simulink model "main"  (R2024b)
settings: Solver=VariableStepAuto  StartTime=0.0  StopTime=0.1  RelTol=1e-3
settings Model: Creator=Admin  LastModifiedBy=Admin

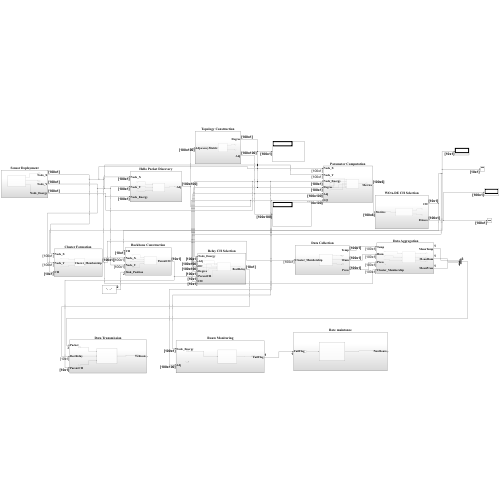
[thumbnail: Simulink's stored preview of the top-level diagram]
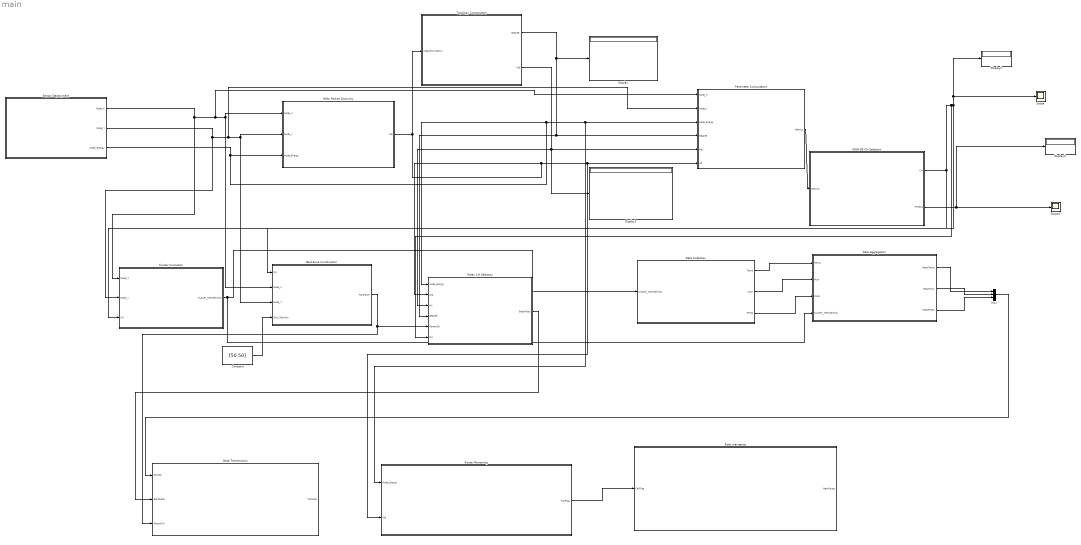
== system main ==
  " Data Aggregation" : Subsystem
  " Data Collection" : Subsystem
  " Route Monitoring" : Subsystem
  Backbone Construction : Subsystem
  Cluster Formation : Subsystem
  Constant : Constant  Value=[50 50]
  Data Transmission : Subsystem
  Display{,1..3} (4 alike) : Display
  Hello Packet Discovery : Subsystem
  Mux : Mux  Inputs=3
  Parameter Computation : Subsystem
  Relay CH Selection : Subsystem
  Rote maintance : Subsystem
  Scope : Scope
  Scope1 : Scope
  Sensor Deployment : Subsystem
  Topology Construction : Subsystem
  WOA-DE CH Selection : Subsystem
  wires:
  Sensor Deployment/2(Node_Y) -> Cluster Formation/2(Node_Y), Parameter Computation/2(Node_Y), Backbone Construction/3(Node_Y), Hello Packet Discovery/2(Node_Y)
  Sensor Deployment/3(Node_Energy) -> Parameter Computation/3(Node_Energy), " Route Monitoring"/1(Node_Energy), Relay CH Selection/1(Node_Energy), Hello Packet Discovery/3(Node_Energy)
  Hello Packet Discovery/1(Adj) -> Parameter Computation/6(LQ), " Route Monitoring"/2(Adj), Relay CH Selection/2(Adj), Topology Construction/1(AdjacencyMatrix)
  Topology Construction/2(Adj) -> Parameter Computation/5(Adj), Relay CH Selection/3(HC), Display1/1
  Sensor Deployment/1(Node_X) -> Cluster Formation/1(Node_X), Backbone Construction/2(Node_X), Hello Packet Discovery/1(Node_X), Parameter Computation/1(Node_X)
  Topology Construction/1(Degree) -> Parameter Computation/4(Degree), Relay CH Selection/4(Degree), Display/1
  Parameter Computation/1(Metrics) -> WOA-DE CH Selection/1(Metrics)
  WOA-DE CH Selection/2(Fitness) -> Display3/1, Scope1/1
  WOA-DE CH Selection/1(CH) -> Relay CH Selection/6(CH), Display2/1, Scope/1, Backbone Construction/1(CH), Cluster Formation/3(CH)
  Constant/1 -> Backbone Construction/4(Sink_Position)
  Backbone Construction/1(ParentCH) -> Data Transmission/3(ParentCH), Relay CH Selection/5(ParentCH)
  Cluster Formation/1(Cluster_Membership) -> " Data Aggregation"/4(Cluster_Membership), " Data Collection"/1(Cluster_Membership)
  " Data Collection"/1(Temp) -> " Data Aggregation"/1(Temp)
  " Data Collection"/2(Hum) -> " Data Aggregation"/2(Hum)
  " Data Collection"/3(Press) -> " Data Aggregation"/3(Press)
  " Data Aggregation"/3(MeanPress) -> Mux/3
  " Data Aggregation"/2(MeanHum) -> Mux/2
  " Data Aggregation"/1(MeanTemp) -> Mux/1
  Mux/1 -> Data Transmission/1(Packet)
  Relay CH Selection/1(BestRelay) -> Data Transmission/2(BestRelay)
  " Route Monitoring"/1(FailFlag) -> Rote maintance/1(FailFlag)

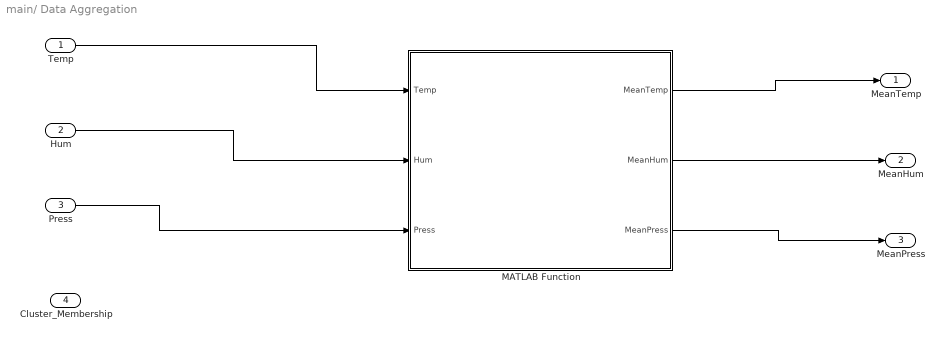
== system main/ Data Aggregation ==
  Temp : Inport
  Hum : Inport  Port=2
  Press : Inport  Port=3
  Cluster_Membership : Inport  Port=4
  MATLAB Function : MATLAB Function  TreatAsAtomicUnit=on
  MeanTemp : Outport
  MeanHum : Outport  Port=2
  MeanPress : Outport  Port=3
  wires:
  Temp/1 -> MATLAB Function/1(Temp)
  Hum/1 -> MATLAB Function/2(Hum)
  Press/1 -> MATLAB Function/3(Press)
  MATLAB Function/1(MeanTemp) -> MeanTemp/1
  MATLAB Function/2(MeanHum) -> MeanHum/1
  MATLAB Function/3(MeanPress) -> MeanPress/1

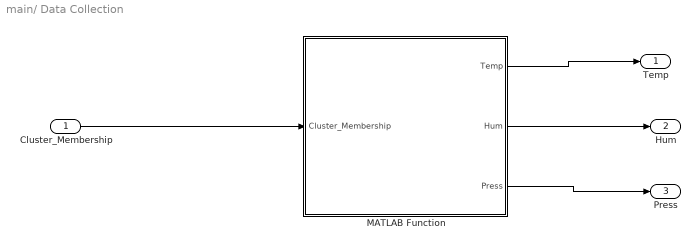
== system main/ Data Collection ==
  Cluster_Membership : Inport
  MATLAB Function : MATLAB Function  TreatAsAtomicUnit=on
  Temp : Outport
  Hum : Outport  Port=2
  Press : Outport  Port=3
  wires:
  Cluster_Membership/1 -> MATLAB Function/1(Cluster_Membership)
  MATLAB Function/1(Temp) -> Temp/1
  MATLAB Function/2(Hum) -> Hum/1
  MATLAB Function/3(Press) -> Press/1

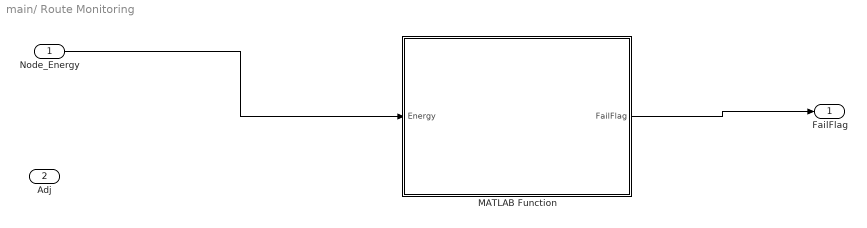
== system main/ Route Monitoring ==
  Node_Energy : Inport
  Adj : Inport  Port=2
  MATLAB Function : MATLAB Function  TreatAsAtomicUnit=on
  FailFlag : Outport
  wires:
  Node_Energy/1 -> MATLAB Function/1(Energy)
  MATLAB Function/1(FailFlag) -> FailFlag/1

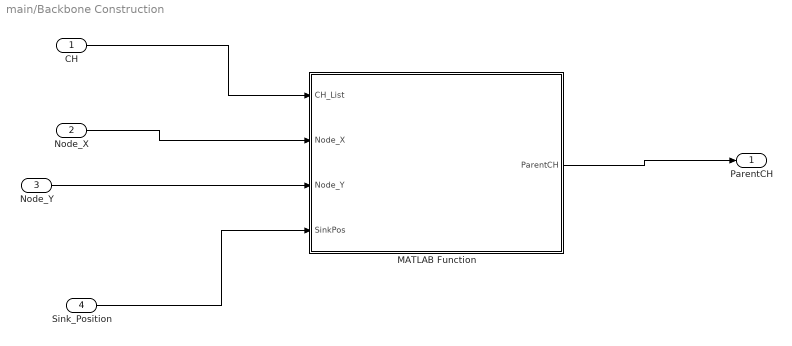
== system main/Backbone Construction ==
  CH : Inport
  Node_X : Inport  Port=2
  Node_Y : Inport  Port=3
  Sink_Position : Inport  Port=4
  MATLAB Function : MATLAB Function  TreatAsAtomicUnit=on
  ParentCH : Outport
  wires:
  CH/1 -> MATLAB Function/1(CH_List)
  Node_X/1 -> MATLAB Function/2(Node_X)
  Node_Y/1 -> MATLAB Function/3(Node_Y)
  Sink_Position/1 -> MATLAB Function/4(SinkPos)
  MATLAB Function/1(ParentCH) -> ParentCH/1

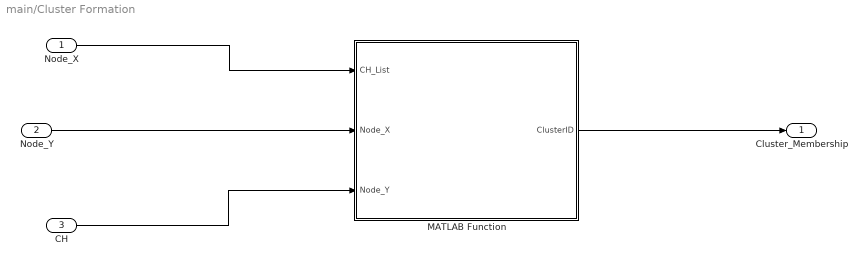
== system main/Cluster Formation ==
  Node_X : Inport
  Node_Y : Inport  Port=2
  CH : Inport  Port=3
  MATLAB Function : MATLAB Function  TreatAsAtomicUnit=on
  Cluster_Membership : Outport
  wires:
  Node_X/1 -> MATLAB Function/1(CH_List)
  Node_Y/1 -> MATLAB Function/2(Node_X)
  CH/1 -> MATLAB Function/3(Node_Y)
  MATLAB Function/1(ClusterID) -> Cluster_Membership/1

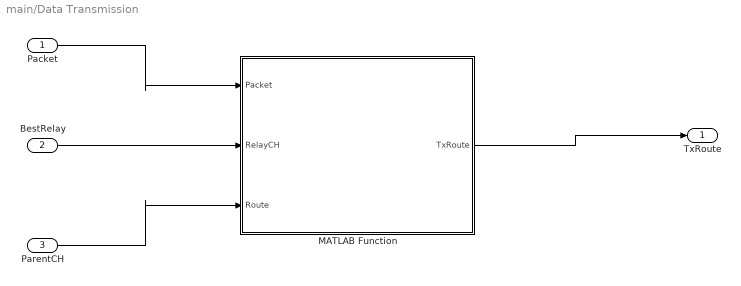
== system main/Data Transmission ==
  Packet : Inport
  BestRelay : Inport  Port=2
  ParentCH : Inport  Port=3
  MATLAB Function : MATLAB Function  TreatAsAtomicUnit=on
  TxRoute : Outport
  wires:
  Packet/1 -> MATLAB Function/1(Packet)
  BestRelay/1 -> MATLAB Function/2(RelayCH)
  ParentCH/1 -> MATLAB Function/3(Route)
  MATLAB Function/1(TxRoute) -> TxRoute/1

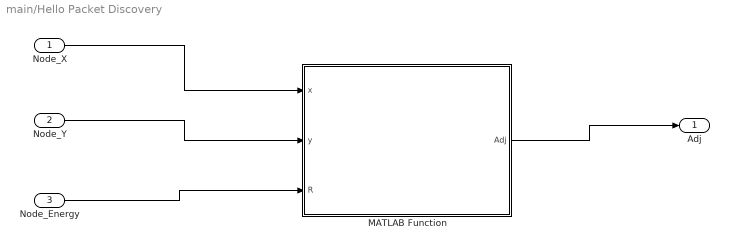
== system main/Hello Packet Discovery ==
  Node_X : Inport
  Node_Y : Inport  Port=2
  Node_Energy : Inport  Port=3
  MATLAB Function : MATLAB Function  TreatAsAtomicUnit=on
  Adj : Outport
  wires:
  Node_X/1 -> MATLAB Function/1(x)
  Node_Y/1 -> MATLAB Function/2(y)
  Node_Energy/1 -> MATLAB Function/3(R)
  MATLAB Function/1(Adj) -> Adj/1

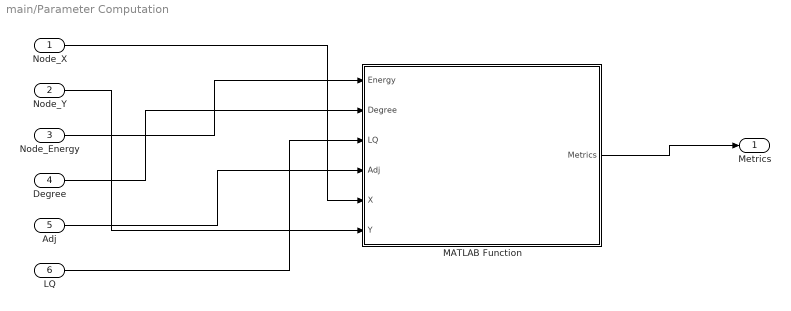
== system main/Parameter Computation ==
  Node_X : Inport
  Node_Y : Inport  Port=2
  Node_Energy : Inport  Port=3
  Degree : Inport  Port=4
  Adj : Inport  Port=5
  LQ : Inport  Port=6
  MATLAB Function : MATLAB Function  TreatAsAtomicUnit=on
  Metrics : Outport
  wires:
  Node_Energy/1 -> MATLAB Function/1(Energy)
  Degree/1 -> MATLAB Function/2(Degree)
  LQ/1 -> MATLAB Function/3(LQ)
  Adj/1 -> MATLAB Function/4(Adj)
  Node_X/1 -> MATLAB Function/5(X)
  Node_Y/1 -> MATLAB Function/6(Y)
  MATLAB Function/1(Metrics) -> Metrics/1

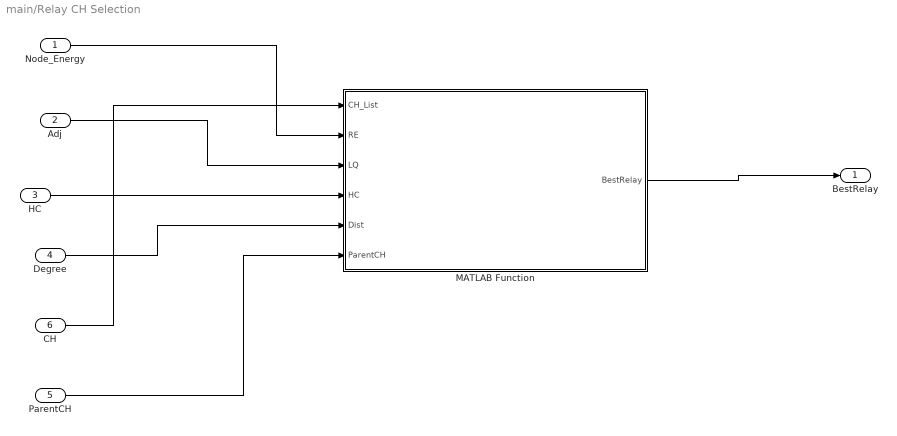
== system main/Relay CH Selection ==
  Node_Energy : Inport
  Adj : Inport  Port=2
  HC : Inport  Port=3
  Degree : Inport  Port=4
  ParentCH : Inport  Port=5
  CH : Inport  Port=6
  MATLAB Function : MATLAB Function  TreatAsAtomicUnit=on
  BestRelay : Outport
  wires:
  Node_Energy/1 -> MATLAB Function/2(RE)
  Adj/1 -> MATLAB Function/3(LQ)
  HC/1 -> MATLAB Function/4(HC)
  Degree/1 -> MATLAB Function/5(Dist)
  CH/1 -> MATLAB Function/1(CH_List)
  ParentCH/1 -> MATLAB Function/6(ParentCH)
  MATLAB Function/1(BestRelay) -> BestRelay/1

== system main/Rote maintance ==
  FailFlag : Inport
  MATLAB Function : MATLAB Function  TreatAsAtomicUnit=on
  NewRoute : Outport
  wires:
  FailFlag/1 -> MATLAB Function/1(FailFlag)
  MATLAB Function/1(NewRoute) -> NewRoute/1

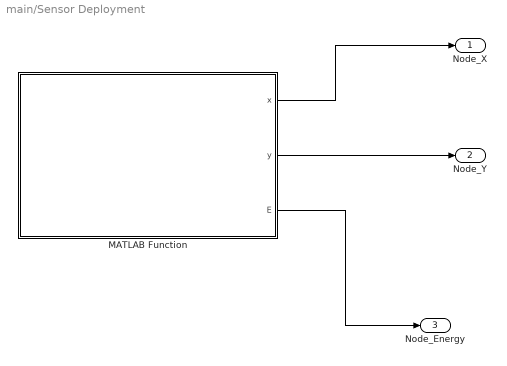
== system main/Sensor Deployment ==
  MATLAB Function : MATLAB Function  TreatAsAtomicUnit=on
  Node_X : Outport
  Node_Y : Outport  Port=2
  Node_Energy : Outport  Port=3
  wires:
  MATLAB Function/1(x) -> Node_X/1
  MATLAB Function/2(y) -> Node_Y/1
  MATLAB Function/3(E) -> Node_Energy/1

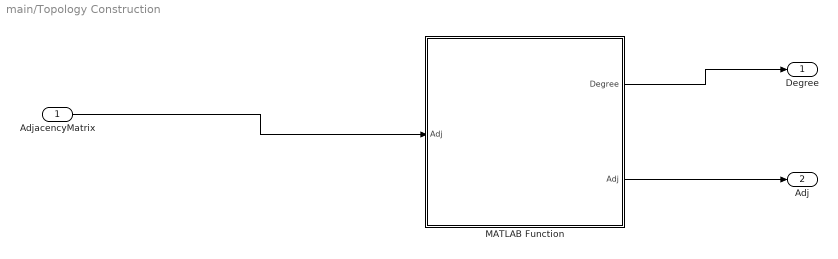
== system main/Topology Construction ==
  AdjacencyMatrix : Inport
  MATLAB Function : MATLAB Function  TreatAsAtomicUnit=on
  Degree : Outport
  Adj : Outport  Port=2
  wires:
  AdjacencyMatrix/1 -> MATLAB Function/1("Adj ")
  MATLAB Function/1(Degree) -> Degree/1
  MATLAB Function/2(Adj) -> Adj/1

== system main/WOA-DE CH Selection ==
  Metrics : Inport
  MATLAB Function : MATLAB Function  TreatAsAtomicUnit=on
  CH : Outport
  Fitness : Outport  Port=2
  wires:
  Metrics/1 -> MATLAB Function/1(Metrics)
  MATLAB Function/1(CH) -> CH/1
  MATLAB Function/2(Fitness) -> Fitness/1

== matlab function main/Data Transmission/MATLAB Function ==
  data: Packet input; TxRoute output; RelayCH input; Route input
function TxRoute = fcn(Packet,RelayCH,Route)

disp('========================');
disp('DATA TRANSMISSION');
disp('========================');

disp('Aggregated Packet Received');

disp(['Relay CH : ' num2str(RelayCH)]);

disp('Transmission Route');

disp(Route);

TxRoute = Route;

end

== matlab function main/ Route Monitoring/MATLAB Function ==
  data: Energy input; FailFlag output
function FailFlag = fcn(Energy)

threshold = 0.2;

if Energy < threshold
    FailFlag = 1;
else
    FailFlag = 0;
end

end

== matlab function main/Hello Packet Discovery/MATLAB Function ==
  data: x input; Adj output; y input; R input
function Adj = fcn(x,y,R)

N = length(x);

Adj = zeros(N,N);

for i = 1:N
    for j = 1:N

        if i ~= j

            d = sqrt((x(i)-x(j))^2 + (y(i)-y(j))^2);

            if d <= R
                Adj(i,j) = 1;
            end

        end

    end
end

end

== matlab function main/Rote maintance/MATLAB Function ==
  data: FailFlag input; NewRoute output
function NewRoute = fcn(FailFlag)

if FailFlag==1

    NewRoute = [43 34];

else

    NewRoute = [75 81 90];

end

end

== matlab function main/Sensor Deployment/MATLAB Function ==
  data: x output; y output; E output
function [x,y,E]=fcn()

N=100;

x=100*rand(N,1);
y=100*rand(N,1);

E=2*ones(N,1);

end

== matlab function main/Topology Construction/MATLAB Function ==
  data: Adj input; Degree output; Adj output
function [Degree,Adj] = TopologyMetrics(Adj)

Degree = sum(Adj,2);

end

== matlab function main/Parameter Computation/MATLAB Function ==
  data: Energy input; Metrics output; Degree input; LQ input; Adj input; X input; Y input
function Metrics = ComputeMetrics(Energy,Degree,LQ,Adj,X,Y)

N = length(Energy);

Metrics = zeros(N,6);

for i = 1:N

    RE = Energy(i);

    ND = Degree(i);

    LinkQ = mean(LQ(i,:));

    HC = 1;    % temporary

    NDen = Degree(i);

    neighbors = find(Adj(i,:)==1);

    if isempty(neighbors)

        AvgDist = 0;

    else

        dist = sqrt((X(i)-X(neighbors)).^2 + ...
                    (Y(i)-Y(neighbors)).^2);

        AvgDist = mean(dist);

    end

    Metrics(i,:) = [RE ND LinkQ HC NDen AvgDist];

end

end

== matlab function main/WOA-DE CH Selection/MATLAB Function ==
  data: Metrics input; CH output; Fitness output
function [CH,Fitness] = FitnessCalculation(Metrics)

N = size(Metrics,1);

Fitness = zeros(N,1);

for i = 1:N

    RE      = Metrics(i,1);
    Degree  = Metrics(i,2);
    LQ      = Metrics(i,3);
    HC      = Metrics(i,4);
    NDen    = Metrics(i,5);
    AvgDist = Metrics(i,6);

    if HC == 0
        HC = 1;
    end

    if AvgDist == 0
        AvgDist = 1;
    end

    Fitness(i) = ...
          0.30*RE ...
        + 0.20*Degree ...
        + 0.20*LQ ...
        + 0.15*NDen ...
        + 0.10*(1/HC) ...
        + 0.05*(1/AvgDist);

end

[~,idx] = sort(Fitness,'descend');

numCH = 10;

CH = idx(1:numCH);

end

== matlab function main/Cluster Formation/MATLAB Function ==
  data: CH_List input; ClusterID output; Node_X input; Node_Y input
function ClusterID = fcn(CH_List,Node_X,Node_Y)

N = length(Node_X);

ClusterID = zeros(N,1);

CHx = Node_X(CH_List);
CHy = Node_Y(CH_List);

for i = 1:N

    dmin = inf;
    bestCH = 1;

    for j = 1:length(CH_List)

        d = sqrt( ...
            (Node_X(i)-CHx(j))^2 + ...
            (Node_Y(i)-CHy(j))^2 );

        if d < dmin

            dmin = d;
            bestCH = CH_List(j);

        end

    end

    ClusterID(i) = bestCH;

end

endfunction y = fcn(u)

y = u;

== matlab function main/Backbone Construction/MATLAB Function ==
  data: CH_List input; ParentCH output; Node_X input; Node_Y input; SinkPos input
function ParentCH = fcn(CH_List,Node_X,Node_Y,SinkPos)

numCH = length(CH_List);

ParentCH = zeros(numCH,1);

sinkX = SinkPos(1);
sinkY = SinkPos(2);

for i = 1:numCH

    currentCH = CH_List(i);

    x1 = Node_X(currentCH);
    y1 = Node_Y(currentCH);

    distSink = sqrt((x1-sinkX)^2 + (y1-sinkY)^2);

    bestParent = 0;
    bestDist = distSink;

    for j = 1:numCH

        if i~=j

            nextCH = CH_List(j);

            x2 = Node_X(nextCH);
            y2 = Node_Y(nextCH);

            d = sqrt((x2-sinkX)^2 + (y2-sinkY)^2);

            if d < bestDist

                bestDist = d;
                bestParent = nextCH;

            end

        end

    end

    ParentCH(i)=bestParent;

end

end

== matlab function main/Relay CH Selection/MATLAB Function ==
  data: CH_List input; BestRelay output; RE input; LQ input; HC input; Dist input; ParentCH input
function BestRelay = fcn(CH_List,RE,LQ,HC,Dist,ParentCH)

numCH = length(CH_List);

BestRelay = zeros(numCH,1);

for i = 1:numCH

    sourceCH = CH_List(i);

    bestFitness = -inf;
    bestRelayCH = sourceCH;

    for j = 1:numCH

        relayCH = CH_List(j);

        if relayCH ~= sourceCH

            fitness = ...
                0.4*RE(relayCH) + ...
                0.3*LQ(relayCH) + ...
                0.2*(1/(HC(relayCH)+1)) + ...
                0.1*(1/(Dist(relayCH)+1));

            if fitness > bestFitness

                bestFitness = fitness;
                bestRelayCH = relayCH;

            end

        end

    end

    BestRelay(i) = bestRelayCH;

end

endfunction y = fcn(u)

y = u;

== matlab function main/ Data Collection/MATLAB Function ==
  data: Temp output; Hum output; Press output; Cluster_Membership input
function [Temp,Hum,Press] = fcn(Cluster_Membership)

N = 100;

Temp  = 25 + 10*rand(N,1);
Hum   = 50 + 20*rand(N,1);
Press = 1000 + 20*rand(N,1);

endfunction y = fcn(u)

y = u;

== matlab function main/ Data Aggregation/MATLAB Function ==
  data: Temp input; MeanTemp output; Hum input; Press input; MeanHum output; MeanPress output
function [MeanTemp,MeanHum,MeanPress] = fcn(Temp,Hum,Press)

MeanTemp = mean(Temp);
MeanHum  = mean(Hum);
MeanPress = mean(Press);

endfunction y = fcn(u)

y = u;
